simulink model "Lab2_Simulink_Design_Part4"  (R2020a)
settings: Solver=VariableStepAuto  StartTime=0.0  StopTime=10.0  RelTol=1e-3
settings Model: Creator=mati1  LastModifiedBy=mati1

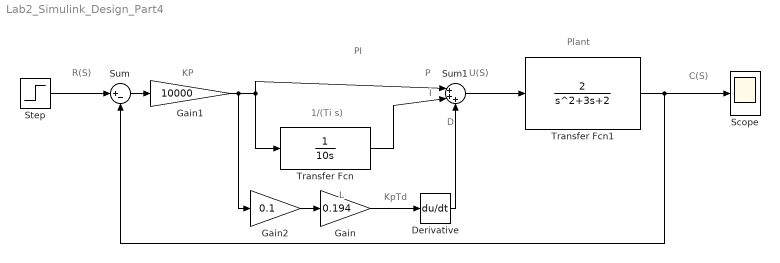
== system Lab2_Simulink_Design_Part4 ==
  note: KpTd
  note: L
  note: I
  note: P
  note: 1/(Ti s)
  note: KP
  note: D
  note: PI
  note: R(S)
  note: C(S)
  note: U(S)
  note: Plant
  Derivative : Derivative
  Gain : Gain  Gain=0.194
  Gain1 : Gain  Gain=10000
  Gain2 : Gain  Gain=0.1
  Scope : Scope
  Step : Step  Before=1  SampleTime=0
  Sum : Sum  Inputs=|+-
  Sum1 : Sum  Inputs=|+++
  Transfer Fcn : TransferFcn  Denominator=[10 0]
  Transfer Fcn1 : TransferFcn  Numerator=[2]  Denominator=[1 3 2]
  wires:
  Step/1 -> Sum/1
  Transfer Fcn1/1 -> Sum/2, Scope/1
  Gain/1 -> Derivative/1
  Sum/1 -> Gain1/1
  Gain1/1 -> Transfer Fcn/1, Sum1/1, Gain2/1
  Derivative/1 -> Sum1/3
  Transfer Fcn/1 -> Sum1/2
  Sum1/1 -> Transfer Fcn1/1
  Gain2/1 -> Gain/1
